simulink model "Sim_Rate_Limiters_simtest"  (Simulink 7.3)
settings: Solver=ode45  StartTime=0.0  StopTime=10.0  RelTol=1e-3
settings Model: Creator=MD710  LastModifiedBy=MD710
settings DebuggingCC: SaveWithParameterizedLinksMsg=none  SolverPrmCheckMsg=none  MultiTaskDSMMsg=warning  MultiTaskCondExecSysMsg=none  FcnCallInpInsideContextMsg=Enable All  StrictBusMsg=None
settings HardwareCC: TargetHWDeviceType=32-bit Generic
settings RTWCC: IncludeERTFirstTime=on
settings GRTTargetCC: TargetFcnLib=ansi_tfl_tmw.mat

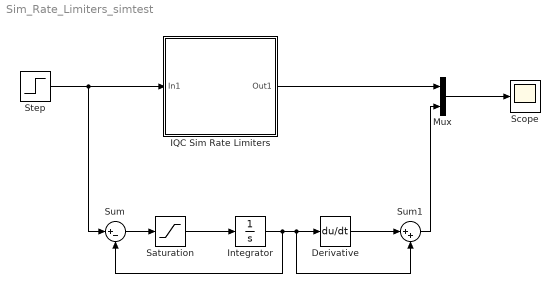
== system Sim_Rate_Limiters_simtest ==
  Derivative : Derivative
  IQC Sim Rate Limiters : Subsystem  mask(IQC Sim Rate Limiters(ver:0.1)){upp_lim=1, low_lim=-1, d_sat=1, firstpole=1, iqc1=on, iqc1_pole=[1], iqc1_out='', iqc2=off, lis_rel=''}
      mask prompts: upp_lim "Upper Limit of Saturation:"; low_lim "Lower Limit of Saturation:"; d_sat "Slope of Saturation:(Default: 1)"; firstpole "(s+Pole1) ~ the Pole1:(Default: 1)"; iqc1 "iqc_ratelimiter(Input,[Pole1 Pole],Slope)  (only for scalar input)"; iqc1_pole "Pole:(Default: [1])"; iqc1_out "Output Variable:(Default: empty)"; iqc2 "Custom IQC"; lis_rel "List of IQC Relationships:"
      mask init:
      | if length(firstpole)>1
      |     error('the Pole1 only scalar')
      | end
      | if length(d_sat)>1
      |     error('d(Sat(0))/dt only scalar')
      | end
      mask Help: <a href="matlab:doc iqc_ratelimiter;">iqc_ratelimiter</a>
      mask CallbackString: ||||iqc_block_cho(gcb,'sim_ratelim_iqc1')|||iqc_block_cho(gcb,'sim_ratelim_iqc2')|
      mask TabNameString: Simulink Parameters,Simulink Parameters,Simulink Parameters,Simulink Parameters,Procedure Parameters,Procedure Parameters,Procedure Parameters,Procedure Parameters,Procedure Parameters
      mask Display: plot(0,0,100,100,[18,45,45,18,18],[60,60,26,26,60],[62,82,82,62,62],[60,60,26,26,60],[62,0],[44,44],[79,65],[44,44],[71,71],[46,57],[68,69,72,74,73,71,69,68,69,72,74],[31,29,29,31,34,35,36,38,40,40,39],[31,31],[26,60],[45,38,24],[55,55,33],[24,18],[33,33],[99,82],[44,44],[10,12,8,10,10,90,90],[44,51,51,44,80,80,44],[7,2],[55,55])
  Integrator : Integrator
  Mux : Mux  Inputs=2
  Saturation : Saturate  UpperLimit=1  LowerLimit=-1
  Scope : Scope
  Step : Step  Time=[2]  SampleTime=0
  Sum : Sum  Inputs=|+-
  Sum1 : Sum  Inputs=|++
  wires:
  Step/1 -> Sum/1, IQC Sim Rate Limiters/1(In1)
  Saturation/1 -> Integrator/1
  Sum/1 -> Saturation/1
  Integrator/1 -> Sum1/2, Derivative/1, Sum/2
  Derivative/1 -> Sum1/1
  IQC Sim Rate Limiters/1(Out1) -> Mux/1
  Sum1/1 -> Mux/2
  Mux/1 -> Scope/1

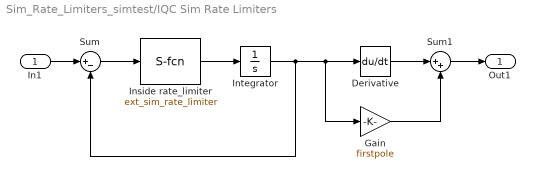
== system Sim_Rate_Limiters_simtest/IQC Sim Rate Limiters ==
  In1 : Inport
  Derivative : Derivative
  Gain : Gain  Gain=firstpole
  Inside rate_limiter : M-S-Function  FunctionName=ext_sim_rate_limiter  Parameters=upp_lim,low_lim,d_sat,firstpole,iqc1,iqc1_pole,iqc1_out,iqc2,lis_rel
  Integrator : Integrator
  Sum : Sum  Inputs=|+-
  Sum1 : Sum  Inputs=|++
  Out1 : Outport
  wires:
  In1/1 -> Sum/1
  Sum1/1 -> Out1/1
  Sum/1 -> Inside rate_limiter/1
  Integrator/1 -> Sum/2, Derivative/1, Gain/1
  Inside rate_limiter/1 -> Integrator/1
  Derivative/1 -> Sum1/1
  Gain/1 -> Sum1/2
